simulink model "multi_gadget"  (Simulink 7.0)
settings: Solver=ode3  SolverMode=SingleTasking  StartTime=0.0  StopTime=Inf  FixedStep=.001  RelTol=1e-3
libraries: xpclib x9, xpcnilib x5, simulink x3, limblab x2, dspsigops x2
settings Model: Creator=Selket  LastModifiedBy=Christian  BufferReuse=off
settings OptimizationCC: BlockReduction=off  OptimizeBlockIOStorage=off  BufferReuse=off  ExpressionFolding=off  LocalBlockOutputs=off
settings DebuggingCC: SaveWithParameterizedLinksMsg=none
settings RTWCC: SystemTargetFile=xpctarget.tlc  TemplateMakefile=xpc_default_tmf  Description=xPC Target  ProcessScript=xpctarget_make_rtw_hook
settings xpcTargetCC: TargetFcnLib=ansi_tfl_tmw.mat  GenFloatMathFcnCalls=ANSI_C  CompOptLevelCompliant=off  PortableWordSizes=off  xPCisDownloadable=off

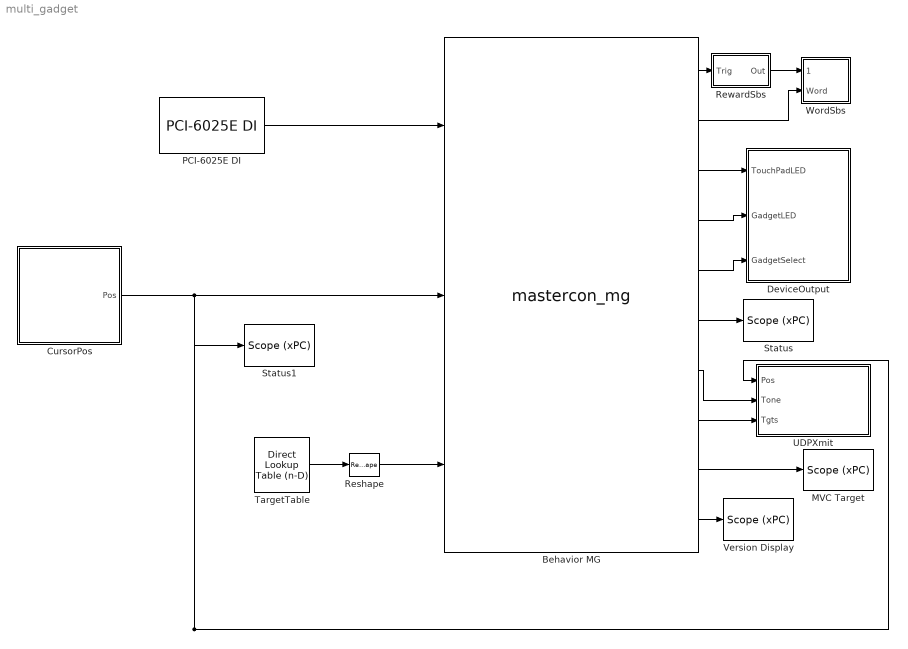
== system multi_gadget ==
  Behavior MG : S-Function  FunctionName=mastercon_mg  Parameters=3 .25 .25 0.5 0.5 5 0.5 1 1 1 0 0 0 0 0 0 0
      mask Display:
      | disp('Master Control\nMulti-Gadget')
      | port_label('input',1,'touch pad')
      | port_label('input',2,'cursor')
      | port_label('input',3,'target list')
      | port_label('output',1,'Reward')
      | port_label('output',2,'Word')
      | port_label('output',3,'TP LED')
      | port_label('output',4,'Gadget LED')
      | port_label('output',5,'Gadget Select')
      | port_label('output',6,'Status')
      | port_label('output',7,'Tone')
      | port_label('output',8,'Targets')
      | port_label('output',9,'MVC Target')
      | port_label('output',10,'Version')
  CursorPos : Subsystem
  DeviceOutput : Subsystem
  MVC Target : xpclib/Misc./Scope (xPC)   SystemSampleTime=-1  scopeno=7  scopetype=Target  autostart=on  viewmode=Numerical  formatstr=' Gadget 1: %6.4f, Gadget 2: %6.4f, Gadget 3: %6.4f, Gadget 4: %6.4f'  grid=on  ylimits=[-10,10]  nosamples=10  noprepostsamples=0  interleave=10  triggermode=FreeRun  triggersignal=1  triggerlevel=0.0  triggerslope=Either  triggerscope=1  triggersample=0  filename=data.dat  mode=Lazy  writesize=512  autorestart=off
  PCI-6025E DI : xpcnilib/Digital Input/PCI-6025E DI  channel=[3]  sampletime=0.001  slot=-1
  Reshape : Reshape  OutputDimensionality=Column vector (2-D)
  RewardSbs : Subsystem
  Status : xpclib/Misc./Scope (xPC)   SystemSampleTime=-1  scopeno=1  scopetype=Target  autostart=on  viewmode=Numerical  formatstr='%6.0f State,%6.0f Rewards,%6.0f Aborts,%6.0f Failures'  grid=on  ylimits=[-10,10]  nosamples=10  noprepostsamples=0  interleave=10  triggermode=FreeRun  triggersignal=1  triggerlevel=0.0  triggerslope=Either  triggerscope=1  triggersample=0  filename=data.dat  mode=Lazy  writesize=512  autorestart=off
  Status1 : xpclib/Misc./Scope (xPC)   SystemSampleTime=-1  scopeno=2  scopetype=Target  autostart=on  viewmode=Numerical  formatstr=' %6.6f X, %6.6f Y'  grid=on  ylimits=[-10,10]  nosamples=10  noprepostsamples=0  interleave=10  triggermode=FreeRun  triggersignal=1  triggerlevel=0.0  triggerslope=Either  triggerscope=1  triggersample=0  filename=data.dat  mode=Lazy  writesize=512  autorestart=off
  TargetTable : simulink/Lookup Tables/Direct Lookup Table (n-D)  maskTabDims=2  explicitNumDims=1  outDims=2-D Matrix  tabIsInput=off  mxTable=[5 5 5 5 5 5 5 5 5 5 5 5 5 5 5 5;5 5 5 5 5 5 5 5 5 5 5 5 5 5 5 5;5 5 5 5 5 5 5 5 5 5 5 5 5 5 5 5;5 5 5 5 5 5 5 5 5 5 5 5 5 5 5 5;5 5 5 5 5 5 5 5 5 5 5 5 5 5 5 5]  clipFlag=Warning  samptime=-1
  UDPXmit : Subsystem
  Version Display : xpclib/Misc./Scope (xPC)   SystemSampleTime=-1  scopeno=5  scopetype=Target  autostart=on  viewmode=Numerical  formatstr='%6.0f major,%6.0f minor,%6.0f revision,%6.0f build'  grid=on  ylimits=[-10,10]  nosamples=10  noprepostsamples=0  interleave=10  triggermode=FreeRun  triggersignal=1  triggerlevel=0.0  triggerslope=Either  triggerscope=1  triggersample=0  filename=data.dat  mode=Lazy  writesize=512  autorestart=off
  WordSbs : Subsystem
  wires:
  Behavior MG/2 -> WordSbs/2(Word)
  Behavior MG/3 -> DeviceOutput/1(TouchPadLED)
  Behavior MG/4 -> DeviceOutput/2(GadgetLED)
  Behavior MG/5 -> DeviceOutput/3(GadgetSelect)
  Behavior MG/6 -> Status/1
  Behavior MG/1 -> RewardSbs/1(Trig)
  Behavior MG/8 -> UDPXmit/3(Tgts)
  PCI-6025E DI/1 -> Behavior MG/1
  TargetTable/1 -> Reshape/1
  CursorPos/1(Pos) -> Behavior MG/2, Status1/1, UDPXmit/1(Pos)
  Behavior MG/7 -> UDPXmit/2(Tone)
  Reshape/1 -> Behavior MG/3
  Behavior MG/9 -> MVC Target/1
  Behavior MG/10 -> Version Display/1
  RewardSbs/1(Out) -> WordSbs/1(Reward)

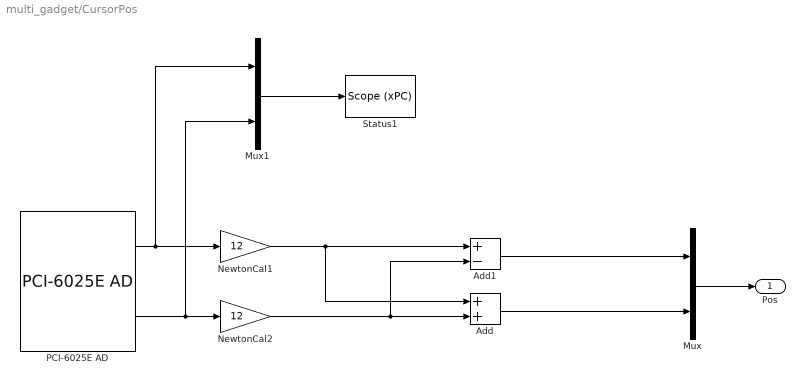
== system multi_gadget/CursorPos ==
  Add : Sum  OutDataType=sfix(16)  OutScaling=2^-10
  Add1 : Sum  Inputs=+-  OutDataType=sfix(16)  OutScaling=2^-10
  Mux : Mux  Inputs=2
  Mux1 : Mux  Inputs=2
  NewtonCal1 : Gain  Gain=12  ParameterDataType=sfix(16)  ParameterScaling=2^0  OutDataType=sfix(16)  OutScaling=2^0
  NewtonCal2 : Gain  Gain=12  ParameterDataType=sfix(16)  ParameterScaling=2^0  OutDataType=sfix(16)  OutScaling=2^0
  PCI-6025E AD : xpcnilib/A//D/PCI-6025E AD  channel=[9 10]  range=[-10]  coupling=[0]  sampletime=0.001  slot=-1
  Status1 : xpclib/Misc./Scope (xPC)   SystemSampleTime=-1  scopeno=4  scopetype=Target  autostart=on  viewmode=Numerical  formatstr=' %6.6f Raw 1, %6.6f Raw 2'  grid=on  ylimits=[-10,10]  nosamples=10  noprepostsamples=0  interleave=10  triggermode=FreeRun  triggersignal=1  triggerlevel=0.0  triggerslope=Either  triggerscope=1  triggersample=0  filename=data.dat  mode=Lazy  writesize=512  autorestart=off
  Pos : Outport  OutDataType=sfix(16)  OutScaling=2^0
  wires:
  PCI-6025E AD/1 -> NewtonCal1/1, Mux1/1
  PCI-6025E AD/2 -> NewtonCal2/1, Mux1/2
  Mux/1 -> Pos/1
  NewtonCal1/1 -> Add/1, Add1/1
  NewtonCal2/1 -> Add/2, Add1/2
  Add/1 -> Mux/2
  Add1/1 -> Mux/1
  Mux1/1 -> Status1/1

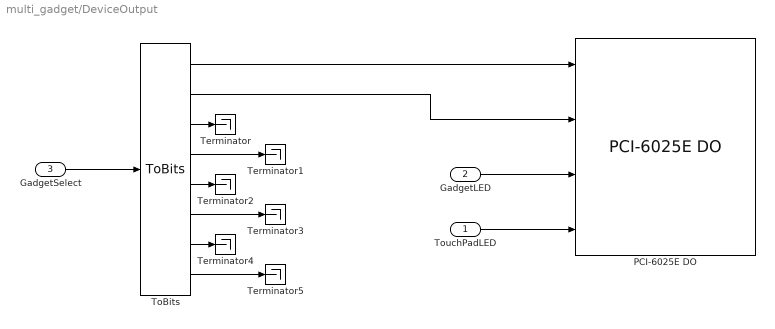
== system multi_gadget/DeviceOutput ==
  TouchPadLED : Inport  OutDataType=sfix(16)  OutScaling=2^0
  GadgetLED : Inport  Port=2  OutDataType=sfix(16)  OutScaling=2^0
  GadgetSelect : Inport  Port=3  OutDataType=sfix(16)  OutScaling=2^0
  PCI-6025E DO : xpcnilib/Digital Output/PCI-6025E DO  channel=[4 5 6 8]  reset=[1]  initValue=[0]  sampletime=0.001  slot=-1
  Terminator{,1..5} (6 alike) : Terminator
  ToBits : limblab/ToBits
  wires:
  GadgetLED/1 -> PCI-6025E DO/3
  TouchPadLED/1 -> PCI-6025E DO/4
  GadgetSelect/1 -> ToBits/1
  ToBits/1 -> PCI-6025E DO/1
  ToBits/2 -> PCI-6025E DO/2
  ToBits/4 -> Terminator1/1
  ToBits/3 -> Terminator/1
  ToBits/5 -> Terminator2/1
  ToBits/6 -> Terminator3/1
  ToBits/7 -> Terminator4/1
  ToBits/8 -> Terminator5/1

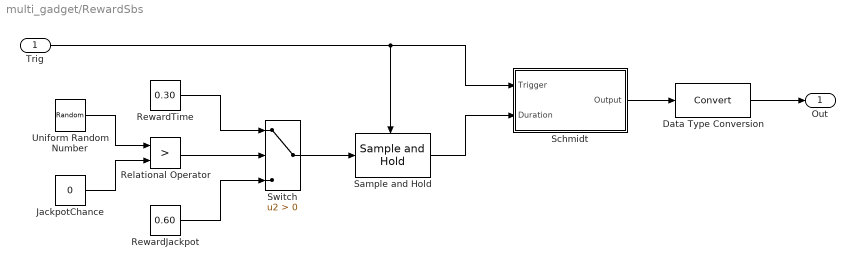
== system multi_gadget/RewardSbs ==
  Trig : Inport  OutDataType=sfix(16)  OutScaling=2^0
  Data Type Conversion : DataTypeConversion  OutDataType=sfix(16)  OutScaling=2^0
  JackpotChance : Constant  Value=0  OutDataType=sfix(16)  OutScaling=2^0
  Relational Operator : RelationalOperator  Operator=>  LogicOutDataTypeMode=boolean
  RewardJackpot : Constant  Value=0.60  OutDataType=sfix(16)  OutScaling=2^0
  RewardTime : Constant  Value=0.30  OutDataType=sfix(16)  OutScaling=2^0
  Sample and Hold : dspsigops/Sample and Hold  SystemSampleTime=-1  trig=Rising edge  initCond=0  latchinput=off
  Schmidt : Subsystem
  Switch : Switch  Criteria=u2 > Threshold  ZeroCross=off
  Uniform Random Number : UniformRandomNumber  Minimum=0  Maximum=100  SampleTime=0.001
  Out : Outport  OutDataType=sfix(16)  OutScaling=2^0
  wires:
  Trig/1 -> Schmidt/1(Trigger), Sample and Hold/Trigger
  Data Type Conversion/1 -> Out/1
  Schmidt/1(Output) -> Data Type Conversion/1
  Sample and Hold/1 -> Schmidt/2(Duration)
  RewardTime/1 -> Switch/1
  RewardJackpot/1 -> Switch/3
  Switch/1 -> Sample and Hold/1
  Uniform Random Number/1 -> Relational Operator/1
  Relational Operator/1 -> Switch/2
  JackpotChance/1 -> Relational Operator/2

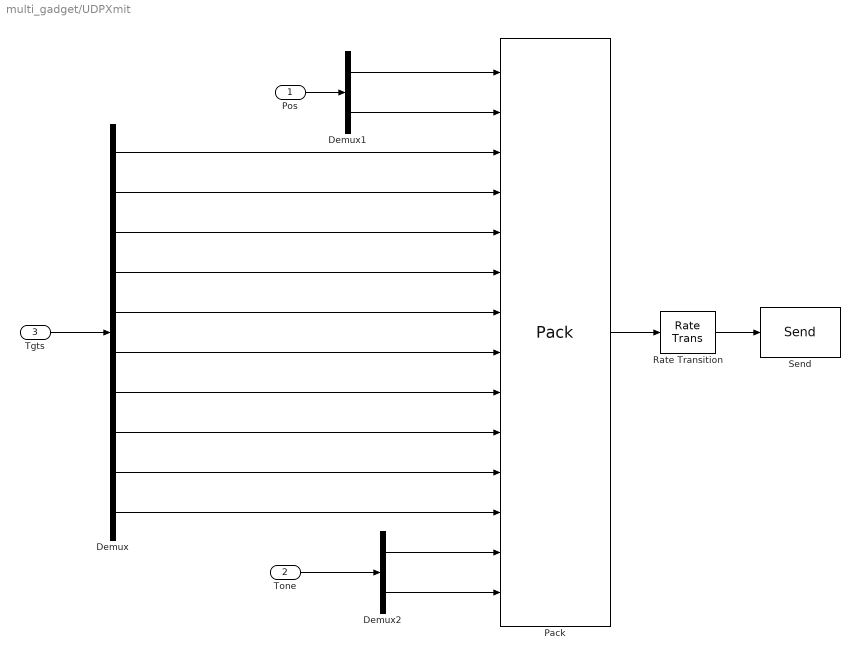
== system multi_gadget/UDPXmit ==
  Pos : Inport  OutDataType=sfix(16)  OutScaling=2^0
  Tone : Inport  Port=2  OutDataType=sfix(16)  OutScaling=2^0
  Tgts : Inport  Port=3  OutDataType=sfix(16)  OutScaling=2^0
  Demux : Demux  Outputs=10
  Demux1 : Demux  Outputs=2
  Demux2 : Demux  Outputs=2
  Pack : xpclib/UDP/Pack  datatypes={'double', 'double','double','double','double','double','double','double','double','double','double','double','double','double'}  byteAlign=1
  Rate Transition : RateTransition
  Send : xpclib/UDP/Send  ipAddress=192.168.0.2  ipPort=25000  localPort=-1  sampletime=.02
  wires:
  Rate Transition/1 -> Send/1
  Pack/1 -> Rate Transition/1
  Demux/10 -> Pack/12
  Demux/9 -> Pack/11
  Demux/8 -> Pack/10
  Demux/7 -> Pack/9
  Demux/6 -> Pack/8
  Demux/5 -> Pack/7
  Demux/4 -> Pack/6
  Demux/3 -> Pack/5
  Demux/2 -> Pack/4
  Demux/1 -> Pack/3
  Demux1/1 -> Pack/1
  Demux1/2 -> Pack/2
  Pos/1 -> Demux1/1
  Demux2/1 -> Pack/13
  Demux2/2 -> Pack/14
  Tone/1 -> Demux2/1
  Tgts/1 -> Demux/1

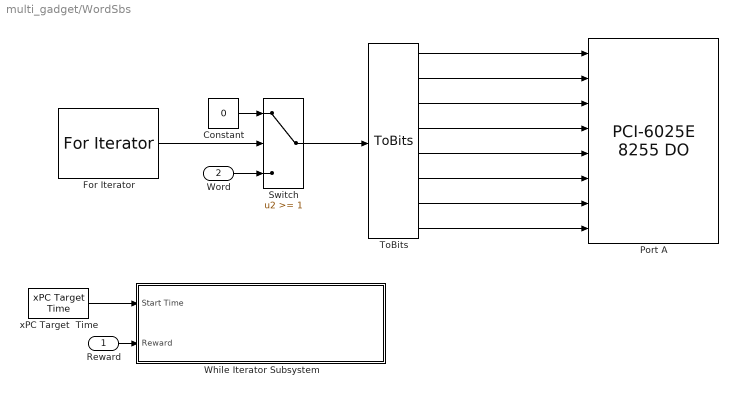
== system multi_gadget/WordSbs ==
  Reward : Inport  OutDataType=sfix(16)  OutScaling=2^0
  Word : Inport  Port=2  OutDataType=sfix(16)  OutScaling=2^0
  Constant : Constant  Value=0  OutDataType=sfix(16)  OutScaling=2^0
  For Iterator : ForIterator  IterationLimit=4  IndexMode=Zero-based  IterationVariableDataType=double
  Port A : xpcnilib/Digital Output/PCI-6025E 8255 DO  channel=1:8  port=A  reset=[1]  initValue=[0]  chip=1  sampletime=-1  slot=-1
  Switch : Switch  Threshold=1  ZeroCross=off
  ToBits : limblab/ToBits
  While Iterator Subsystem : Subsystem  TreatAsAtomicUnit=on
  "xPC Target  Time " : xpclib/Misc./xPC Target  Time   ts=-1
  wires:
  ToBits/1 -> Port A/1
  ToBits/2 -> Port A/2
  ToBits/3 -> Port A/3
  ToBits/4 -> Port A/4
  ToBits/5 -> Port A/5
  ToBits/6 -> Port A/6
  ToBits/7 -> Port A/7
  ToBits/8 -> Port A/8
  For Iterator/1 -> Switch/2
  Constant/1 -> Switch/1
  Word/1 -> Switch/3
  Switch/1 -> ToBits/1
  "xPC Target  Time "/1 -> While Iterator Subsystem/1(Start Time)
  Reward/1 -> While Iterator Subsystem/2(Reward)

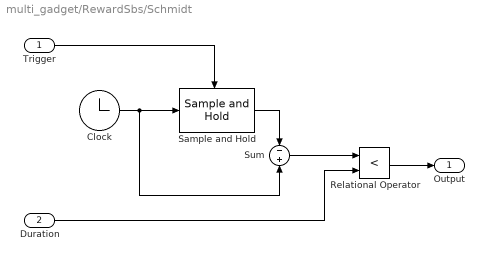
== system multi_gadget/RewardSbs/Schmidt ==
  Trigger : Inport  OutDataType=sfix(16)  OutScaling=2^0
  Duration : Inport  Port=2  OutDataType=sfix(16)  OutScaling=2^0
  Clock : Clock
  Relational Operator : RelationalOperator  Operator=<  LogicOutDataTypeMode=boolean
  Sample and Hold : dspsigops/Sample and Hold  SystemSampleTime=-1  trig=Rising edge  initCond=-1000  latchinput=off
  Sum : Sum  Inputs=-+  OutDataType=sfix(16)  OutScaling=2^0
  Output : Outport  OutDataType=sfix(16)  OutScaling=2^0
  wires:
  Clock/1 -> Sum/2, Sample and Hold/1
  Sample and Hold/1 -> Sum/1
  Sum/1 -> Relational Operator/1
  Duration/1 -> Relational Operator/2
  Relational Operator/1 -> Output/1
  Trigger/1 -> Sample and Hold/Trigger

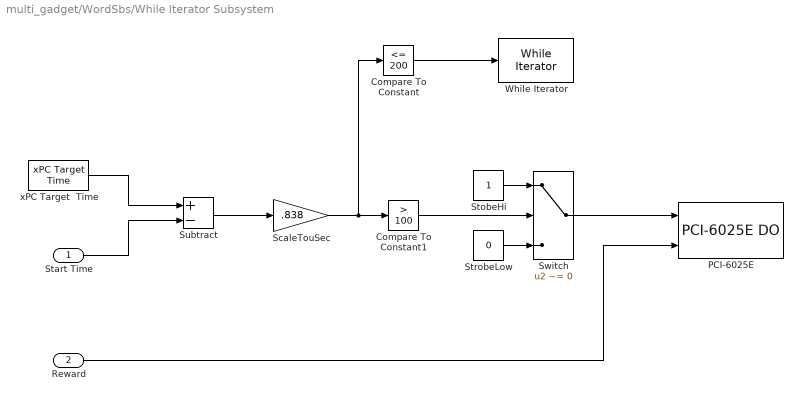
== system multi_gadget/WordSbs/While Iterator Subsystem ==
  Start Time : Inport  OutDataType=sfix(16)  OutScaling=2^0
  Reward : Inport  Port=2  OutDataType=sfix(16)  OutScaling=2^0
  Compare To Constant : simulink/Logic and Bit Operations/Compare To Constant  SystemSampleTime=-1  relop=<=  const=200  LogicOutDataTypeMode=boolean
  Compare To Constant1 : simulink/Logic and Bit Operations/Compare To Constant  SystemSampleTime=-1  relop=>  const=100  LogicOutDataTypeMode=boolean  ZeroCross=off
  "PCI-6025E " : xpcnilib/Digital Output/PCI-6025E DO  channel=[1 2]  reset=[1]  initValue=[0]  sampletime=-1  slot=-1
  ScaleTouSec : Gain  Gain=.838  ParameterDataType=sfix(16)  ParameterScaling=2^0  OutDataType=sfix(16)  OutScaling=2^0
  StobeHi : Constant  OutDataType=sfix(16)  OutScaling=2^0
  StrobeLow : Constant  Value=0  OutDataType=sfix(16)  OutScaling=2^0
  Subtract : Sum  Inputs=+-  OutDataType=sfix(16)  OutScaling=2^-10
  Switch : Switch  Criteria=u2 ~= 0
  While Iterator : WhileIterator  MaxIters=-1  WhileBlockType=do-while
  "xPC Target  Time " : xpclib/Misc./xPC Target  Time   ts=-1
  wires:
  "xPC Target  Time "/1 -> Subtract/1
  Start Time/1 -> Subtract/2
  Subtract/1 -> ScaleTouSec/1
  Compare To Constant/1 -> While Iterator/1
  ScaleTouSec/1 -> Compare To Constant/1, Compare To Constant1/1
  Compare To Constant1/1 -> Switch/2
  StobeHi/1 -> Switch/1
  StrobeLow/1 -> Switch/3
  Switch/1 -> "PCI-6025E "/1
  Reward/1 -> "PCI-6025E "/2
